simulink model "W01_Base_Map_cs"  (R2019a)
settings: Solver=FixedStepDiscrete  StartTime=0.0  StopTime=40  FixedStep=1/20  RelTol=1e-3
PreLoadFcn:
  | mbxruntime.callbacks.PreLoadFcn(bdroot);
  | check_NUTS_defined
  | model_closed = 0;
  | assignin('base',['model_closed_' bdroot],false);
PostLoadFcn:
  | mbxruntime.callbacks.PostLoadFcn(bdroot);
InitFcn:
  | mbxruntime.callbacks.InitFcn(bdroot);
StartFcn:
  | mbxruntime.callbacks.StartFcn(bdroot);
StopFcn:
  | mbxruntime.callbacks.StopFcn(bdroot);;
  | 
model workspace: external: MAT-File .\W01_Base_Map_cs_hws.mat (data not in the file)
undefined symbols (not defined in the file or in its folder): DiscIntNeverNeededParam, InitImageOutputDir, mbxruntime, tabledata, W01_Base_Map_cs_328ec7e3a8cd5b54, W01_Base_Map_cs_423c72fa17799c7f, W01_Base_Map_cs_514c2dea2cdbe680, W01_Base_Map_cs_51d6e6e467bedba1, W01_Base_Map_cs_563ebd29d1fd6c09, W01_Base_Map_cs_57ea59d0358dab77, W01_Base_Map_cs_669d1acb174df2b9, W01_Base_Map_cs_774a522413284ef7, W01_Base_Map_cs_9538d35a279fbe4e, W01_Base_Map_cs_9f504bb84aebc2fd, W01_Base_Map_cs_a242ed7539861165, W01_Base_Map_cs_ae41b72d7e14f81d, W01_Base_Map_cs_Audi_A8_Sedan_1_Path_pathUniqueID, W01_Base_Map_cs_b5931a786e299506, W01_Base_Map_cs_b7f45a070fa6e639, W01_Base_Map_cs_c02beb48492dde12, W01_Base_Map_cs_c75b75e9f6b035bf, W01_Base_Map_cs_cf83ac8e8b053cbf, W01_Base_Map_cs_Child_RegularAni_1_Path_pathUniqueID, W01_Base_Map_cs_Child_RegularAni_2_Path_pathUniqueID, W01_Base_Map_cs_Citroen_C3_Hatchback_1_Path_pathUniqueID, W01_Base_Map_cs_d4423fcf1c0d6fc4, W01_Base_Map_cs_df133aa86d9852fe, W01_Base_Map_cs_Female_RegularAni_1_Path_pathUniqueID, W01_Base_Map_cs_Male_RegularAni_1_Path_pathUniqueID, W01_Base_Map_cs_Male_RegularAni_2_Path_pathUniqueID
libraries: simulink_extras x41, adeye_lib x15, simulink x10, dspindex x6, PreScanSimulinkLibrary x4, sharedtransform x3, robotcorelib x1, PreScanUsefulBlocks x1
(part 10 of 11)

== system W01_Base_Map_cs/TrafficLightRoadSideNL_6/Orange_Mux ==
  MSCD [Cd] : Inport
  Position (xyz) [m] : Inport  Port=2
  Orientation (RPY) [deg] : Inport  Port=3
  Color [-] : Inport  Port=4
  TextureResourceID [-] : Inport  Port=5
  Bus Creator : BusCreator  Inputs='Intensity','Position','Orientation','Color','TextureResourceID'  OutDataTypeStr=Bus: PRESCAN_VISULIGHTACTUATOR_DATA  NonVirtualBus=on
  Bus Creator1 : BusCreator  Inputs=3  OutDataTypeStr=Bus: PRESCAN_RGB_DATA  NonVirtualBus=on
  Bus Creator2 : BusCreator  Inputs=3  OutDataTypeStr=Bus: PRESCAN_RPY_DATA  NonVirtualBus=on
  Bus Creator3 : BusCreator  Inputs=3  OutDataTypeStr=Bus: PRESCAN_XYZ_DATA  NonVirtualBus=on
  Data Type Conversion : DataTypeConversion  OutDataTypeStr=int32  RndMeth=Nearest
  Degrees to Radians : simulink_extras/Transformations/Degrees to Radians
  Demux : Demux  Outputs=3
  Demux1 : Demux  Outputs=3
  Demux2 : Demux  Outputs=3
  Lights : Outport
  wires:
  TextureResourceID [-]/1 -> Data Type Conversion/1  "TextureResourceID"
  MSCD [Cd]/1 -> Bus Creator/1  "Intensity"
  Bus Creator/1 -> Lights/1
  Demux/1 -> Bus Creator1/1  "R"
  Demux/2 -> Bus Creator1/2  "G"
  Demux/3 -> Bus Creator1/3  "B"
  Color [-]/1 -> Demux/1  "Color"
  Bus Creator1/1 -> Bus Creator/4  "Color"
  Demux1/1 -> Bus Creator2/1  "Roll"
  Demux1/2 -> Bus Creator2/2  "Pitch"
  Demux1/3 -> Bus Creator2/3  "Yaw"
  Orientation (RPY) [deg]/1 -> Degrees to Radians/1  "Orientation"
  Bus Creator2/1 -> Bus Creator/3  "Orientation"
  Demux2/1 -> Bus Creator3/1  "X"
  Demux2/2 -> Bus Creator3/2  "Y"
  Demux2/3 -> Bus Creator3/3  "Z"
  Position (xyz) [m]/1 -> Demux2/1  "Position"
  Bus Creator3/1 -> Bus Creator/2  "Position"
  Data Type Conversion/1 -> Bus Creator/5  "TextureResourceID"
  Degrees to Radians/1 -> Demux1/1

== system W01_Base_Map_cs/TrafficLightRoadSideNL_6/Red_Mux ==
  MSCD [Cd] : Inport
  Position (xyz) [m] : Inport  Port=2
  Orientation (RPY) [deg] : Inport  Port=3
  Color [-] : Inport  Port=4
  TextureResourceID [-] : Inport  Port=5
  Bus Creator : BusCreator  Inputs='Intensity','Position','Orientation','Color','TextureResourceID'  OutDataTypeStr=Bus: PRESCAN_VISULIGHTACTUATOR_DATA  NonVirtualBus=on
  Bus Creator1 : BusCreator  Inputs=3  OutDataTypeStr=Bus: PRESCAN_RGB_DATA  NonVirtualBus=on
  Bus Creator2 : BusCreator  Inputs=3  OutDataTypeStr=Bus: PRESCAN_RPY_DATA  NonVirtualBus=on
  Bus Creator3 : BusCreator  Inputs=3  OutDataTypeStr=Bus: PRESCAN_XYZ_DATA  NonVirtualBus=on
  Data Type Conversion : DataTypeConversion  OutDataTypeStr=int32  RndMeth=Nearest
  Degrees to Radians : simulink_extras/Transformations/Degrees to Radians
  Demux : Demux  Outputs=3
  Demux1 : Demux  Outputs=3
  Demux2 : Demux  Outputs=3
  Lights : Outport
  wires:
  TextureResourceID [-]/1 -> Data Type Conversion/1  "TextureResourceID"
  MSCD [Cd]/1 -> Bus Creator/1  "Intensity"
  Bus Creator/1 -> Lights/1
  Demux/1 -> Bus Creator1/1  "R"
  Demux/2 -> Bus Creator1/2  "G"
  Demux/3 -> Bus Creator1/3  "B"
  Color [-]/1 -> Demux/1  "Color"
  Bus Creator1/1 -> Bus Creator/4  "Color"
  Demux1/1 -> Bus Creator2/1  "Roll"
  Demux1/2 -> Bus Creator2/2  "Pitch"
  Demux1/3 -> Bus Creator2/3  "Yaw"
  Orientation (RPY) [deg]/1 -> Degrees to Radians/1  "Orientation"
  Bus Creator2/1 -> Bus Creator/3  "Orientation"
  Demux2/1 -> Bus Creator3/1  "X"
  Demux2/2 -> Bus Creator3/2  "Y"
  Demux2/3 -> Bus Creator3/3  "Z"
  Position (xyz) [m]/1 -> Demux2/1  "Position"
  Bus Creator3/1 -> Bus Creator/2  "Position"
  Data Type Conversion/1 -> Bus Creator/5  "TextureResourceID"
  Degrees to Radians/1 -> Demux1/1

== system W01_Base_Map_cs/TrafficLightRoadSideNL_7/Green_Mux ==
  MSCD [Cd] : Inport
  Position (xyz) [m] : Inport  Port=2
  Orientation (RPY) [deg] : Inport  Port=3
  Color [-] : Inport  Port=4
  TextureResourceID [-] : Inport  Port=5
  Bus Creator : BusCreator  Inputs='Intensity','Position','Orientation','Color','TextureResourceID'  OutDataTypeStr=Bus: PRESCAN_VISULIGHTACTUATOR_DATA  NonVirtualBus=on
  Bus Creator1 : BusCreator  Inputs=3  OutDataTypeStr=Bus: PRESCAN_RGB_DATA  NonVirtualBus=on
  Bus Creator2 : BusCreator  Inputs=3  OutDataTypeStr=Bus: PRESCAN_RPY_DATA  NonVirtualBus=on
  Bus Creator3 : BusCreator  Inputs=3  OutDataTypeStr=Bus: PRESCAN_XYZ_DATA  NonVirtualBus=on
  Data Type Conversion : DataTypeConversion  OutDataTypeStr=int32  RndMeth=Nearest
  Degrees to Radians : simulink_extras/Transformations/Degrees to Radians
  Demux : Demux  Outputs=3
  Demux1 : Demux  Outputs=3
  Demux2 : Demux  Outputs=3
  Lights : Outport
  wires:
  TextureResourceID [-]/1 -> Data Type Conversion/1  "TextureResourceID"
  MSCD [Cd]/1 -> Bus Creator/1  "Intensity"
  Bus Creator/1 -> Lights/1
  Demux/1 -> Bus Creator1/1  "R"
  Demux/2 -> Bus Creator1/2  "G"
  Demux/3 -> Bus Creator1/3  "B"
  Color [-]/1 -> Demux/1  "Color"
  Bus Creator1/1 -> Bus Creator/4  "Color"
  Demux1/1 -> Bus Creator2/1  "Roll"
  Demux1/2 -> Bus Creator2/2  "Pitch"
  Demux1/3 -> Bus Creator2/3  "Yaw"
  Orientation (RPY) [deg]/1 -> Degrees to Radians/1  "Orientation"
  Bus Creator2/1 -> Bus Creator/3  "Orientation"
  Demux2/1 -> Bus Creator3/1  "X"
  Demux2/2 -> Bus Creator3/2  "Y"
  Demux2/3 -> Bus Creator3/3  "Z"
  Position (xyz) [m]/1 -> Demux2/1  "Position"
  Bus Creator3/1 -> Bus Creator/2  "Position"
  Data Type Conversion/1 -> Bus Creator/5  "TextureResourceID"
  Degrees to Radians/1 -> Demux1/1

== system W01_Base_Map_cs/TrafficLightRoadSideNL_7/Orange_Mux ==
  MSCD [Cd] : Inport
  Position (xyz) [m] : Inport  Port=2
  Orientation (RPY) [deg] : Inport  Port=3
  Color [-] : Inport  Port=4
  TextureResourceID [-] : Inport  Port=5
  Bus Creator : BusCreator  Inputs='Intensity','Position','Orientation','Color','TextureResourceID'  OutDataTypeStr=Bus: PRESCAN_VISULIGHTACTUATOR_DATA  NonVirtualBus=on
  Bus Creator1 : BusCreator  Inputs=3  OutDataTypeStr=Bus: PRESCAN_RGB_DATA  NonVirtualBus=on
  Bus Creator2 : BusCreator  Inputs=3  OutDataTypeStr=Bus: PRESCAN_RPY_DATA  NonVirtualBus=on
  Bus Creator3 : BusCreator  Inputs=3  OutDataTypeStr=Bus: PRESCAN_XYZ_DATA  NonVirtualBus=on
  Data Type Conversion : DataTypeConversion  OutDataTypeStr=int32  RndMeth=Nearest
  Degrees to Radians : simulink_extras/Transformations/Degrees to Radians
  Demux : Demux  Outputs=3
  Demux1 : Demux  Outputs=3
  Demux2 : Demux  Outputs=3
  Lights : Outport
  wires:
  TextureResourceID [-]/1 -> Data Type Conversion/1  "TextureResourceID"
  MSCD [Cd]/1 -> Bus Creator/1  "Intensity"
  Bus Creator/1 -> Lights/1
  Demux/1 -> Bus Creator1/1  "R"
  Demux/2 -> Bus Creator1/2  "G"
  Demux/3 -> Bus Creator1/3  "B"
  Color [-]/1 -> Demux/1  "Color"
  Bus Creator1/1 -> Bus Creator/4  "Color"
  Demux1/1 -> Bus Creator2/1  "Roll"
  Demux1/2 -> Bus Creator2/2  "Pitch"
  Demux1/3 -> Bus Creator2/3  "Yaw"
  Orientation (RPY) [deg]/1 -> Degrees to Radians/1  "Orientation"
  Bus Creator2/1 -> Bus Creator/3  "Orientation"
  Demux2/1 -> Bus Creator3/1  "X"
  Demux2/2 -> Bus Creator3/2  "Y"
  Demux2/3 -> Bus Creator3/3  "Z"
  Position (xyz) [m]/1 -> Demux2/1  "Position"
  Bus Creator3/1 -> Bus Creator/2  "Position"
  Data Type Conversion/1 -> Bus Creator/5  "TextureResourceID"
  Degrees to Radians/1 -> Demux1/1

== system W01_Base_Map_cs/TrafficLightRoadSideNL_7/Red_Mux ==
  MSCD [Cd] : Inport
  Position (xyz) [m] : Inport  Port=2
  Orientation (RPY) [deg] : Inport  Port=3
  Color [-] : Inport  Port=4
  TextureResourceID [-] : Inport  Port=5
  Bus Creator : BusCreator  Inputs='Intensity','Position','Orientation','Color','TextureResourceID'  OutDataTypeStr=Bus: PRESCAN_VISULIGHTACTUATOR_DATA  NonVirtualBus=on
  Bus Creator1 : BusCreator  Inputs=3  OutDataTypeStr=Bus: PRESCAN_RGB_DATA  NonVirtualBus=on
  Bus Creator2 : BusCreator  Inputs=3  OutDataTypeStr=Bus: PRESCAN_RPY_DATA  NonVirtualBus=on
  Bus Creator3 : BusCreator  Inputs=3  OutDataTypeStr=Bus: PRESCAN_XYZ_DATA  NonVirtualBus=on
  Data Type Conversion : DataTypeConversion  OutDataTypeStr=int32  RndMeth=Nearest
  Degrees to Radians : simulink_extras/Transformations/Degrees to Radians
  Demux : Demux  Outputs=3
  Demux1 : Demux  Outputs=3
  Demux2 : Demux  Outputs=3
  Lights : Outport
  wires:
  TextureResourceID [-]/1 -> Data Type Conversion/1  "TextureResourceID"
  MSCD [Cd]/1 -> Bus Creator/1  "Intensity"
  Bus Creator/1 -> Lights/1
  Demux/1 -> Bus Creator1/1  "R"
  Demux/2 -> Bus Creator1/2  "G"
  Demux/3 -> Bus Creator1/3  "B"
  Color [-]/1 -> Demux/1  "Color"
  Bus Creator1/1 -> Bus Creator/4  "Color"
  Demux1/1 -> Bus Creator2/1  "Roll"
  Demux1/2 -> Bus Creator2/2  "Pitch"
  Demux1/3 -> Bus Creator2/3  "Yaw"
  Orientation (RPY) [deg]/1 -> Degrees to Radians/1  "Orientation"
  Bus Creator2/1 -> Bus Creator/3  "Orientation"
  Demux2/1 -> Bus Creator3/1  "X"
  Demux2/2 -> Bus Creator3/2  "Y"
  Demux2/3 -> Bus Creator3/3  "Z"
  Position (xyz) [m]/1 -> Demux2/1  "Position"
  Bus Creator3/1 -> Bus Creator/2  "Position"
  Data Type Conversion/1 -> Bus Creator/5  "TextureResourceID"
  Degrees to Radians/1 -> Demux1/1

== system W01_Base_Map_cs/TrafficLightRoadSideNL_8/Green_Mux ==
  MSCD [Cd] : Inport
  Position (xyz) [m] : Inport  Port=2
  Orientation (RPY) [deg] : Inport  Port=3
  Color [-] : Inport  Port=4
  TextureResourceID [-] : Inport  Port=5
  Bus Creator : BusCreator  Inputs='Intensity','Position','Orientation','Color','TextureResourceID'  OutDataTypeStr=Bus: PRESCAN_VISULIGHTACTUATOR_DATA  NonVirtualBus=on
  Bus Creator1 : BusCreator  Inputs=3  OutDataTypeStr=Bus: PRESCAN_RGB_DATA  NonVirtualBus=on
  Bus Creator2 : BusCreator  Inputs=3  OutDataTypeStr=Bus: PRESCAN_RPY_DATA  NonVirtualBus=on
  Bus Creator3 : BusCreator  Inputs=3  OutDataTypeStr=Bus: PRESCAN_XYZ_DATA  NonVirtualBus=on
  Data Type Conversion : DataTypeConversion  OutDataTypeStr=int32  RndMeth=Nearest
  Degrees to Radians : simulink_extras/Transformations/Degrees to Radians
  Demux : Demux  Outputs=3
  Demux1 : Demux  Outputs=3
  Demux2 : Demux  Outputs=3
  Lights : Outport
  wires:
  TextureResourceID [-]/1 -> Data Type Conversion/1  "TextureResourceID"
  MSCD [Cd]/1 -> Bus Creator/1  "Intensity"
  Bus Creator/1 -> Lights/1
  Demux/1 -> Bus Creator1/1  "R"
  Demux/2 -> Bus Creator1/2  "G"
  Demux/3 -> Bus Creator1/3  "B"
  Color [-]/1 -> Demux/1  "Color"
  Bus Creator1/1 -> Bus Creator/4  "Color"
  Demux1/1 -> Bus Creator2/1  "Roll"
  Demux1/2 -> Bus Creator2/2  "Pitch"
  Demux1/3 -> Bus Creator2/3  "Yaw"
  Orientation (RPY) [deg]/1 -> Degrees to Radians/1  "Orientation"
  Bus Creator2/1 -> Bus Creator/3  "Orientation"
  Demux2/1 -> Bus Creator3/1  "X"
  Demux2/2 -> Bus Creator3/2  "Y"
  Demux2/3 -> Bus Creator3/3  "Z"
  Position (xyz) [m]/1 -> Demux2/1  "Position"
  Bus Creator3/1 -> Bus Creator/2  "Position"
  Data Type Conversion/1 -> Bus Creator/5  "TextureResourceID"
  Degrees to Radians/1 -> Demux1/1

== system W01_Base_Map_cs/TrafficLightRoadSideNL_8/Orange_Mux ==
  MSCD [Cd] : Inport
  Position (xyz) [m] : Inport  Port=2
  Orientation (RPY) [deg] : Inport  Port=3
  Color [-] : Inport  Port=4
  TextureResourceID [-] : Inport  Port=5
  Bus Creator : BusCreator  Inputs='Intensity','Position','Orientation','Color','TextureResourceID'  OutDataTypeStr=Bus: PRESCAN_VISULIGHTACTUATOR_DATA  NonVirtualBus=on
  Bus Creator1 : BusCreator  Inputs=3  OutDataTypeStr=Bus: PRESCAN_RGB_DATA  NonVirtualBus=on
  Bus Creator2 : BusCreator  Inputs=3  OutDataTypeStr=Bus: PRESCAN_RPY_DATA  NonVirtualBus=on
  Bus Creator3 : BusCreator  Inputs=3  OutDataTypeStr=Bus: PRESCAN_XYZ_DATA  NonVirtualBus=on
  Data Type Conversion : DataTypeConversion  OutDataTypeStr=int32  RndMeth=Nearest
  Degrees to Radians : simulink_extras/Transformations/Degrees to Radians
  Demux : Demux  Outputs=3
  Demux1 : Demux  Outputs=3
  Demux2 : Demux  Outputs=3
  Lights : Outport
  wires:
  TextureResourceID [-]/1 -> Data Type Conversion/1  "TextureResourceID"
  MSCD [Cd]/1 -> Bus Creator/1  "Intensity"
  Bus Creator/1 -> Lights/1
  Demux/1 -> Bus Creator1/1  "R"
  Demux/2 -> Bus Creator1/2  "G"
  Demux/3 -> Bus Creator1/3  "B"
  Color [-]/1 -> Demux/1  "Color"
  Bus Creator1/1 -> Bus Creator/4  "Color"
  Demux1/1 -> Bus Creator2/1  "Roll"
  Demux1/2 -> Bus Creator2/2  "Pitch"
  Demux1/3 -> Bus Creator2/3  "Yaw"
  Orientation (RPY) [deg]/1 -> Degrees to Radians/1  "Orientation"
  Bus Creator2/1 -> Bus Creator/3  "Orientation"
  Demux2/1 -> Bus Creator3/1  "X"
  Demux2/2 -> Bus Creator3/2  "Y"
  Demux2/3 -> Bus Creator3/3  "Z"
  Position (xyz) [m]/1 -> Demux2/1  "Position"
  Bus Creator3/1 -> Bus Creator/2  "Position"
  Data Type Conversion/1 -> Bus Creator/5  "TextureResourceID"
  Degrees to Radians/1 -> Demux1/1

== system W01_Base_Map_cs/TrafficLightRoadSideNL_8/Red_Mux ==
  MSCD [Cd] : Inport
  Position (xyz) [m] : Inport  Port=2
  Orientation (RPY) [deg] : Inport  Port=3
  Color [-] : Inport  Port=4
  TextureResourceID [-] : Inport  Port=5
  Bus Creator : BusCreator  Inputs='Intensity','Position','Orientation','Color','TextureResourceID'  OutDataTypeStr=Bus: PRESCAN_VISULIGHTACTUATOR_DATA  NonVirtualBus=on
  Bus Creator1 : BusCreator  Inputs=3  OutDataTypeStr=Bus: PRESCAN_RGB_DATA  NonVirtualBus=on
  Bus Creator2 : BusCreator  Inputs=3  OutDataTypeStr=Bus: PRESCAN_RPY_DATA  NonVirtualBus=on
  Bus Creator3 : BusCreator  Inputs=3  OutDataTypeStr=Bus: PRESCAN_XYZ_DATA  NonVirtualBus=on
  Data Type Conversion : DataTypeConversion  OutDataTypeStr=int32  RndMeth=Nearest
  Degrees to Radians : simulink_extras/Transformations/Degrees to Radians
  Demux : Demux  Outputs=3
  Demux1 : Demux  Outputs=3
  Demux2 : Demux  Outputs=3
  Lights : Outport
  wires:
  TextureResourceID [-]/1 -> Data Type Conversion/1  "TextureResourceID"
  MSCD [Cd]/1 -> Bus Creator/1  "Intensity"
  Bus Creator/1 -> Lights/1
  Demux/1 -> Bus Creator1/1  "R"
  Demux/2 -> Bus Creator1/2  "G"
  Demux/3 -> Bus Creator1/3  "B"
  Color [-]/1 -> Demux/1  "Color"
  Bus Creator1/1 -> Bus Creator/4  "Color"
  Demux1/1 -> Bus Creator2/1  "Roll"
  Demux1/2 -> Bus Creator2/2  "Pitch"
  Demux1/3 -> Bus Creator2/3  "Yaw"
  Orientation (RPY) [deg]/1 -> Degrees to Radians/1  "Orientation"
  Bus Creator2/1 -> Bus Creator/3  "Orientation"
  Demux2/1 -> Bus Creator3/1  "X"
  Demux2/2 -> Bus Creator3/2  "Y"
  Demux2/3 -> Bus Creator3/3  "Z"
  Position (xyz) [m]/1 -> Demux2/1  "Position"
  Bus Creator3/1 -> Bus Creator/2  "Position"
  Data Type Conversion/1 -> Bus Creator/5  "TextureResourceID"
  Degrees to Radians/1 -> Demux1/1

== system W01_Base_Map_cs/pose_otheCar/PoseArray Publisher ==
  seq : Inport
  frameId : Inport  Port=2
  frameId_length : Inport  Port=3
  poses : Inport  Port=4
  poses_length : Inport  Port=5
  seq1 : Inport  Port=6
  frameId1 : Inport  Port=7
  frameId_length1 : Inport  Port=8
  poses1 : Inport  Port=9
  poses_length1 : Inport  Port=10
  seq2 : Inport  Port=11
  frameId2 : Inport  Port=12
  frameId_length2 : Inport  Port=13
  poses2 : Inport  Port=14
  poses_length2 : Inport  Port=15
  Demux : Demux  Outputs=7
  Demux1 : Demux  Outputs=7
  Demux2 : Demux  Outputs=7
  S-Function Builder : S-Function  InitFcn=try, set_param(gcb,'FunctionName','PoseArray3_publisher'), end  FunctionName=PoseArray3_publisher  Parameters=int8(topic),int8(message_type),port,timeout  SFunctionModules=PoseArray3_publisher_wrapper rosbridge_functions  SFunctionDeploymentMode=off  EnableBusSupport=off  mask(S-Function Builder){}
      mask help: Simulink:masks:SFunctionBuilder_MD
      mask init:
      | val = [[.9  0.75 0.75 1 1 .9 .9 1]',[1 1 0.75 0.75 .9 .9 1 .9]'];try , sys = get_param(gcb,'SfunBuilderFcnName');if isempty(sys), sys = get_param(gcb,'FunctionName'); end,catch, sys = get_param(gcb,'FunctionName'); end
      settings: CopyFcn=set_param(gcbh,'LinkStatus','none')  PreSaveFcn=try, set_param(gcb,'FunctionName','PoseArray3_publisher'), end  OpenFcn=sfunctionwizard(gcbh)
      mask Display: plot(val(:,1),val(:,2)),disp(sys), port_label('input',1,'seq'), port_label('input',2,'frameId'), port_label('input',3,'frameId_length'), port_label('input',4,'positionX'), port_label('input',5,'positionY'), port_label('input',6,'positionZ'), port_label('input',7,'orientationW'), port_label('input',8,'orientationX'), port_label('input',9,'orientationY'), port_label('input',10,'orientationZ'), port_label('input',11,'poses_length'), port_label('input',12,'seq1'), port_label('input',13,'frameId1'), port_label('input',14,'frameId_length1'), port_label('input',15,'positionX1'), port_label('input',16,'positionY1'), port_label('input',17,'positionZ1'), port_label('input',18,'orientationW1'), port_label('input',19,'orientationX1'), port_label('input',20,'orientationY1'), port_label('input',21,'orientationZ1'), port_label('input',22,'poses_length1'), port_label('input',23,'seq2'), port_label('input',24,'frameId2'), port_label('input',25,'frameId_length2'), port_label('input',26,'positionX2'), port_label('input',27,'positionY2'), port_label('input',28,'positionZ2'), port_label('input',29,'orientationW2'), port_label('input',30,'orientationX2'), port_label('input',31,'orientationY2'), port_label('input',32,'orientationZ2'), port_label('input',33,'poses_length2')
  wires:
  seq/1 -> S-Function Builder/1
  Demux/1 -> S-Function Builder/4
  Demux/2 -> S-Function Builder/5
  Demux/3 -> S-Function Builder/6
  Demux/4 -> S-Function Builder/7
  Demux/5 -> S-Function Builder/8
  Demux/6 -> S-Function Builder/9
  Demux/7 -> S-Function Builder/10
  frameId_length/1 -> S-Function Builder/3
  frameId/1 -> S-Function Builder/2
  poses/1 -> Demux/1
  poses_length/1 -> S-Function Builder/11
  frameId1/1 -> S-Function Builder/13
  frameId_length1/1 -> S-Function Builder/14
  seq1/1 -> S-Function Builder/12
  Demux1/6 -> S-Function Builder/20
  Demux1/2 -> S-Function Builder/16
  Demux1/7 -> S-Function Builder/21
  Demux1/5 -> S-Function Builder/19
  Demux1/3 -> S-Function Builder/17
  Demux1/4 -> S-Function Builder/18
  Demux1/1 -> S-Function Builder/15
  poses1/1 -> Demux1/1
  poses_length1/1 -> S-Function Builder/22
  seq2/1 -> S-Function Builder/23
  frameId2/1 -> S-Function Builder/24
  frameId_length2/1 -> S-Function Builder/25
  Demux2/6 -> S-Function Builder/31
  Demux2/4 -> S-Function Builder/29
  Demux2/3 -> S-Function Builder/28
  Demux2/2 -> S-Function Builder/27
  Demux2/7 -> S-Function Builder/32
  poses2/1 -> Demux2/1
  Demux2/1 -> S-Function Builder/26
  Demux2/5 -> S-Function Builder/30
  poses_length2/1 -> S-Function Builder/33

== system W01_Base_Map_cs/Audi_A8_Sedan_1/SELF_Demux/compas converter ==
  rotz [rad] : Inport
  cart2compas : Subsystem
  rad2deg : Gain  Gain=180/pi
  heading [deg] : Outport
  wires:
  rad2deg/1 -> cart2compas/1(Angle [deg])
  rotz [rad]/1 -> rad2deg/1
  cart2compas/1(heading [deg]) -> heading [deg]/1

== system W01_Base_Map_cs/BMW_X5_SUV_1/Dynamics_Empty/MuxState ==
  note: mode: Dynamics
  note: mode: Positioning
  note: mode: Dynamics
      | VelVEHICLE
      | wrt VEH
  note: AnglesVEHICLE
      | wrtGLOB
  note: For state mode 'Dynamic' positions
      | are not taken into account, as they
      | are computed by integrating velocity.
      | Click annotation for Help.
  x [m] : Inport  SampleTime=TimeStep
  y [m] : Inport  Port=2  SampleTime=TimeStep
  z [m] : Inport  Port=3  SampleTime=TimeStep
  dx [m/s] : Inport  Port=4  SampleTime=TimeStep
  dy [m/s] : Inport  Port=5  SampleTime=TimeStep
  dz [m/s] : Inport  Port=6  SampleTime=TimeStep
  R [rad] : Inport  Port=7  SampleTime=TimeStep
  P [rad] : Inport  Port=8  SampleTime=TimeStep
  Y [rad] : Inport  Port=9  SampleTime=TimeStep
  Constant : Constant  DisableCoverage=on  Value=positioningmode
  Discrete-Time Integrator : DiscreteIntegrator  SampleTime=TimeStep  ICPrevOutput=DiscIntNeverNeededParam  ICPrevScaledInput=DiscIntNeverNeededParam
  Ground : Ground
  Ground1 : Ground
  Mux1 : Mux  Inputs=[3 3]
  Mux2 : Mux  Inputs=3
  Mux3 : Mux  Inputs=3
  Mux4 : Mux  Inputs=3
  Mux5 : Mux  Inputs=[3 3]
  Mux6 : Mux  Inputs=[6 3]
  Switch : Switch  Threshold=0.5
  Transformation_BODY2GLOBAL : PreScanSimulinkLibrary/Simple_Vehicle_Dynamics/Chassis/MuxDynState/Transformation_BODY2GLOBAL  SystemSampleTime=-1
  mux3 : Mux  Inputs=3
  state : Outport
  wires:
  Constant/1 -> Switch/2
  Mux6/1 -> state/1
  Mux4/1 -> Mux1/1
  Mux5/1 -> Switch/3
  Mux1/1 -> Switch/1
  Switch/1 -> Mux6/1  "PosVeh wrt  GLOB"
  P [rad]/1 -> Mux3/2
  R [rad]/1 -> Mux3/1
  dz [m/s]/1 -> Mux2/3
  dy [m/s]/1 -> Mux2/2
  dx [m/s]/1 -> Mux2/1
  z [m]/1 -> Mux4/3
  y [m]/1 -> Mux4/2
  x [m]/1 -> Mux4/1
  Ground1/1 -> mux3/2  "pitch"
  Y [rad]/1 -> mux3/3, Mux3/3  "yaw"
  Mux3/1 -> Mux6/2
  Transformation_BODY2GLOBAL/1 -> Discrete-Time Integrator/1, Mux5/2  "VelVEH wrt  GLOB"
  mux3/1 -> Transformation_BODY2GLOBAL/2
  Ground/1 -> mux3/1  "roll"
  Mux2/1 -> Mux1/2, Transformation_BODY2GLOBAL/1
  Discrete-Time Integrator/1 -> Mux5/1  "PosVEH wrt  GLOB"

== system W01_Base_Map_cs/BMW_X5_SUV_1/Dynamics_Empty/STATE_BMW_X5_SUV_1 ==
  State : Inport  SampleTime=TimeStep
  Bus Creator : BusCreator  Inputs=15  OutDataTypeStr=Bus: PRESCAN_STATEACTUATORDATA  NonVirtualBus=on
  Constant : Constant  Value=0
  Demux : Demux  Outputs=15
  Mux : Mux  Inputs=3
  Mux1 : Mux  Inputs=3
  Mux2 : Mux  Inputs=3
  iniBODYAngles wrtVEH [rad] : Constant  Value=Roll0  SampleTime=TimeStep
  iniBODYAngles wrtVEH [rad]1 : Constant  Value=Pitch0  SampleTime=TimeStep
  iniVEHAngles wrtGLOB [rad] : Constant  Value=Yaw0  SampleTime=TimeStep
  iniVEHposition wrtGLOB [m] : Constant  Value=x0  SampleTime=TimeStep
  iniVEHposition wrtGLOB [m]1 : Constant  Value=y0  SampleTime=TimeStep
  iniVEHposition wrtGLOB [m]2 : Constant  Value=z0  SampleTime=TimeStep
  state2FullState : PreScanSimulinkLibrary/state2FullState  SystemSampleTime=-1
  StateBus : Outport  OutDataTypeStr=Bus: PRESCAN_STATEACTUATORDATA
  wires:
  Mux2/1 -> state2FullState/4
  iniVEHAngles wrtGLOB [rad]/1 -> Mux2/3
  Mux1/1 -> state2FullState/3
  Constant/1 -> Mux2/1, Mux2/2, Mux1/3
  iniBODYAngles wrtVEH [rad]1/1 -> Mux1/2
  iniBODYAngles wrtVEH [rad]/1 -> Mux1/1
  Mux/1 -> state2FullState/2
  iniVEHposition wrtGLOB [m]2/1 -> Mux/3
  iniVEHposition wrtGLOB [m]/1 -> Mux/1
  iniVEHposition wrtGLOB [m]1/1 -> Mux/2
  Demux/15 -> Bus Creator/15  "AngularVelocityYaw"
  Demux/14 -> Bus Creator/14  "AngularVelocityPitch"
  Demux/13 -> Bus Creator/13  "AngularVelocityRoll"
  Demux/12 -> Bus Creator/12  "OrientationYaw"
  Demux/11 -> Bus Creator/11  "OrientationPitch"
  Demux/10 -> Bus Creator/10  "OrientationRoll"
  Demux/9 -> Bus Creator/9  "AccelerationZ"
  Demux/8 -> Bus Creator/8  "AccelerationY"
  Demux/7 -> Bus Creator/7  "AccelerationX"
  Demux/6 -> Bus Creator/6  "VelocityZ"
  Demux/5 -> Bus Creator/5  "VelocityY"
  Demux/4 -> Bus Creator/4  "VelocityX"
  Demux/3 -> Bus Creator/3  "PositionZ"
  Demux/2 -> Bus Creator/2  "PositionY"
  Demux/1 -> Bus Creator/1  "PositionX"
  state2FullState/1 -> Demux/1
  State/1 -> state2FullState/1
  Bus Creator/1 -> StateBus/1

== system W01_Base_Map_cs/BMW_X5_SUV_1/Dynamics_Empty/Subsystem1 ==
  note: For state mode 'Dynamic' positions
      | are not taken into account, as they
      | are computed by integrating velocity.
      | Click annotation for Help.
  In1 : Inport
  Data Type Conversion{6..11} (6 alike) : DataTypeConversion
  Discrete-Time Integrator4 : DiscreteIntegrator  SampleTime=-1  ICPrevOutput=DiscIntNeverNeededParam  ICPrevScaledInput=DiscIntNeverNeededParam
  Discrete-Time Integrator5 : DiscreteIntegrator  SampleTime=-1  ICPrevOutput=DiscIntNeverNeededParam  ICPrevScaledInput=DiscIntNeverNeededParam
  Discrete-Time Integrator6 : DiscreteIntegrator  SampleTime=-1  ICPrevOutput=DiscIntNeverNeededParam  ICPrevScaledInput=DiscIntNeverNeededParam
  Subsystem : Subsystem
  TwistStamped Subscriber : Subsystem  mask{topic='/TwistS', message_type='geometry_msgs/TwistStamped', port=9090, timeout=2}
      mask prompts: topic "Topic name"; message_type "Message type"; timeout "Timeout (s)"
  Out1 : Outport
  Out2 : Outport  Port=2
  Out3 : Outport  Port=3
  Out4 : Outport  Port=4
  Out5 : Outport  Port=5
  Out6 : Outport  Port=6
  wires:
  Discrete-Time Integrator6/1 -> Out4/1
  In1/1 -> Subsystem/1(In1)
  Subsystem/1(Out1) -> Out1/1
  Data Type Conversion8/1 -> Out3/1
  Discrete-Time Integrator4/1 -> Out6/1
  Data Type Conversion7/1 -> Out2/1
  Discrete-Time Integrator5/1 -> Out5/1
  Data Type Conversion9/1 -> Discrete-Time Integrator6/1
  Data Type Conversion10/1 -> Discrete-Time Integrator5/1
  Data Type Conversion11/1 -> Discrete-Time Integrator4/1
  Data Type Conversion6/1 -> Subsystem/2(In2)
  TwistStamped Subscriber/1(linear_x) -> Data Type Conversion6/1
  TwistStamped Subscriber/2(linear_y) -> Data Type Conversion7/1
  TwistStamped Subscriber/3(linear_z) -> Data Type Conversion8/1
  TwistStamped Subscriber/4(angular_x) -> Data Type Conversion9/1
  TwistStamped Subscriber/5(angular_y) -> Data Type Conversion10/1
  TwistStamped Subscriber/6(angular_z) -> Data Type Conversion11/1

== system W01_Base_Map_cs/BMW_X5_SUV_1/Fault Injection Camera1/If Action Subsystem ==
  In1 : Inport
  In2 : Inport  Port=2
  In3 : Inport  Port=3
  Action Port : ActionPort
  Out1 : Outport
  Out2 : Outport  Port=2
  Out3 : Outport  Port=3
  wires:
  In1/1 -> Out1/1
  In2/1 -> Out2/1
  In3/1 -> Out3/1

== system W01_Base_Map_cs/BMW_X5_SUV_1/Fault Injection Camera1/If Action Subsystem1 ==
  In2 : Inport
  In3 : Inport  Port=2
  In4 : Inport  Port=3
  In5 : Inport  Port=4
  In6 : Inport  Port=5
  In7 : Inport  Port=6
  Action Port : ActionPort
  Assignment1 : Assignment  NumberOfDimensions=2  DiagnosticForDimensions=Warning  IndexOptions=Starting index (port),Starting index (port)  Indices=1,1  OutputSizes=1000,1
  Assignment2 : Assignment  NumberOfDimensions=2  DiagnosticForDimensions=Warning  IndexOptions=Starting index (port),Starting index (port)  Indices=1,1  OutputSizes=1000,1
  Assignment3 : Assignment  NumberOfDimensions=2  DiagnosticForDimensions=Warning  IndexOptions=Starting index (port),Starting index (port)  Indices=1,1  OutputSizes=1000,1
  Out2 : Outport
  Out3 : Outport  Port=2
  Out4 : Outport  Port=3
  wires:
  In2/1 -> Assignment3/3, Assignment1/3, Assignment2/3
  In6/1 -> Assignment1/1
  Assignment1/1 -> Out3/1
  In4/1 -> Assignment3/2, Assignment1/2, Assignment2/2
  Assignment2/1 -> Out2/1
  Assignment3/1 -> Out4/1
  In7/1 -> Assignment3/1
  In5/1 -> Assignment2/1
  In3/1 -> Assignment2/4, Assignment1/4, Assignment3/4

== system W01_Base_Map_cs/BMW_X5_SUV_1/Fault Injection Listener Camera 1/Int16 Subscriber ==
  S-Function Builder : S-Function  InitFcn=try, set_param(gcb,'FunctionName','int16_subscriber'), end  FunctionName=int16_subscriber  Parameters=int8(topic),int8(message_type),port,timeout  SFunctionModules=int16_subscriber_wrapper rosbridge_functions  SFunctionDeploymentMode=off  EnableBusSupport=off  mask(S-Function Builder){}
      mask help: Simulink:masks:SFunctionBuilder_MD
      mask init: same as W01_Base_Map_cs/pose_otheCar/PoseArray Publisher/S-Function Builder
      settings: CopyFcn=set_param(gcbh,'LinkStatus','none')  PreSaveFcn=try, set_param(gcb,'FunctionName','int16_subscriber'), end  OpenFcn=sfunctionwizard(gcbh)
      mask Display: plot(val(:,1),val(:,2)),disp(sys), port_label('output',1,'data')
  data : Outport
  wires:
  S-Function Builder/1 -> data/1

== system W01_Base_Map_cs/BMW_X5_SUV_1/Fault Injection Listener Camera 2/Int16 Subscriber ==
  S-Function Builder : S-Function  InitFcn=try, set_param(gcb,'FunctionName','int16_subscriber'), end  FunctionName=int16_subscriber  Parameters=int8(topic),int8(message_type),port,timeout  SFunctionModules=int16_subscriber_wrapper rosbridge_functions  SFunctionDeploymentMode=off  EnableBusSupport=off  mask(S-Function Builder){}
      mask help: Simulink:masks:SFunctionBuilder_MD
      mask init: same as W01_Base_Map_cs/pose_otheCar/PoseArray Publisher/S-Function Builder
      settings: CopyFcn=set_param(gcbh,'LinkStatus','none')  PreSaveFcn=try, set_param(gcb,'FunctionName','int16_subscriber'), end  OpenFcn=sfunctionwizard(gcbh)
      mask Display: plot(val(:,1),val(:,2)),disp(sys), port_label('output',1,'data')
  data : Outport
  wires:
  S-Function Builder/1 -> data/1

== system W01_Base_Map_cs/BMW_X5_SUV_1/Fault Injection Listener GNSS/Int16 Subscriber ==
  S-Function Builder : S-Function  InitFcn=try, set_param(gcb,'FunctionName','int16_subscriber'), end  FunctionName=int16_subscriber  Parameters=int8(topic),int8(message_type),port,timeout  SFunctionModules=int16_subscriber_wrapper rosbridge_functions  SFunctionDeploymentMode=off  EnableBusSupport=off  mask(S-Function Builder){}
      mask help: Simulink:masks:SFunctionBuilder_MD
      mask init: same as W01_Base_Map_cs/pose_otheCar/PoseArray Publisher/S-Function Builder
      settings: CopyFcn=set_param(gcbh,'LinkStatus','none')  PreSaveFcn=try, set_param(gcb,'FunctionName','int16_subscriber'), end  OpenFcn=sfunctionwizard(gcbh)
      mask Display: plot(val(:,1),val(:,2)),disp(sys), port_label('output',1,'data')
  data : Outport
  wires:
  S-Function Builder/1 -> data/1

== system W01_Base_Map_cs/BMW_X5_SUV_1/Fault Injection Listener Lidar 1/Int16 Subscriber ==
  S-Function Builder : S-Function  InitFcn=try, set_param(gcb,'FunctionName','int16_subscriber'), end  FunctionName=int16_subscriber  Parameters=int8(topic),int8(message_type),port,timeout  SFunctionModules=int16_subscriber_wrapper rosbridge_functions  SFunctionDeploymentMode=off  EnableBusSupport=off  mask(S-Function Builder){}
      mask help: Simulink:masks:SFunctionBuilder_MD
      mask init: same as W01_Base_Map_cs/pose_otheCar/PoseArray Publisher/S-Function Builder
      settings: CopyFcn=set_param(gcbh,'LinkStatus','none')  PreSaveFcn=try, set_param(gcb,'FunctionName','int16_subscriber'), end  OpenFcn=sfunctionwizard(gcbh)
      mask Display: plot(val(:,1),val(:,2)),disp(sys), port_label('output',1,'data')
  data : Outport
  wires:
  S-Function Builder/1 -> data/1

== system W01_Base_Map_cs/BMW_X5_SUV_1/Fault Injection Listener Lidar 2/Int16 Subscriber ==
  S-Function Builder : S-Function  InitFcn=try, set_param(gcb,'FunctionName','int16_subscriber'), end  FunctionName=int16_subscriber  Parameters=int8(topic),int8(message_type),port,timeout  SFunctionModules=int16_subscriber_wrapper rosbridge_functions  SFunctionDeploymentMode=off  EnableBusSupport=off  mask(S-Function Builder){}
      mask help: Simulink:masks:SFunctionBuilder_MD
      mask init: same as W01_Base_Map_cs/pose_otheCar/PoseArray Publisher/S-Function Builder
      settings: CopyFcn=set_param(gcbh,'LinkStatus','none')  PreSaveFcn=try, set_param(gcb,'FunctionName','int16_subscriber'), end  OpenFcn=sfunctionwizard(gcbh)
      mask Display: plot(val(:,1),val(:,2)),disp(sys), port_label('output',1,'data')
  data : Outport
  wires:
  S-Function Builder/1 -> data/1

== system W01_Base_Map_cs/BMW_X5_SUV_1/Fault Injection Listener Lidar 3/Int16 Subscriber ==
  S-Function Builder : S-Function  InitFcn=try, set_param(gcb,'FunctionName','int16_subscriber'), end  FunctionName=int16_subscriber  Parameters=int8(topic),int8(message_type),port,timeout  SFunctionModules=int16_subscriber_wrapper rosbridge_functions  SFunctionDeploymentMode=off  EnableBusSupport=off  mask(S-Function Builder){}
      mask help: Simulink:masks:SFunctionBuilder_MD
      mask init: same as W01_Base_Map_cs/pose_otheCar/PoseArray Publisher/S-Function Builder
      settings: CopyFcn=set_param(gcbh,'LinkStatus','none')  PreSaveFcn=try, set_param(gcb,'FunctionName','int16_subscriber'), end  OpenFcn=sfunctionwizard(gcbh)
      mask Display: plot(val(:,1),val(:,2)),disp(sys), port_label('output',1,'data')
  data : Outport
  wires:
  S-Function Builder/1 -> data/1

== system W01_Base_Map_cs/BMW_X5_SUV_1/Fault Injection Listener Lidar 4/Int16 Subscriber ==
  S-Function Builder : S-Function  InitFcn=try, set_param(gcb,'FunctionName','int16_subscriber'), end  FunctionName=int16_subscriber  Parameters=int8(topic),int8(message_type),port,timeout  SFunctionModules=int16_subscriber_wrapper rosbridge_functions  SFunctionDeploymentMode=off  EnableBusSupport=off  mask(S-Function Builder){}
      mask help: Simulink:masks:SFunctionBuilder_MD
      mask init: same as W01_Base_Map_cs/pose_otheCar/PoseArray Publisher/S-Function Builder
      settings: CopyFcn=set_param(gcbh,'LinkStatus','none')  PreSaveFcn=try, set_param(gcb,'FunctionName','int16_subscriber'), end  OpenFcn=sfunctionwizard(gcbh)
      mask Display: plot(val(:,1),val(:,2)),disp(sys), port_label('output',1,'data')
  data : Outport
  wires:
  S-Function Builder/1 -> data/1

== system W01_Base_Map_cs/BMW_X5_SUV_1/Fault Injection Listener Radar/Int16 Subscriber ==
  S-Function Builder : S-Function  InitFcn=try, set_param(gcb,'FunctionName','int16_subscriber'), end  FunctionName=int16_subscriber  Parameters=int8(topic),int8(message_type),port,timeout  SFunctionModules=int16_subscriber_wrapper rosbridge_functions  SFunctionDeploymentMode=off  EnableBusSupport=off  mask(S-Function Builder){}
      mask help: Simulink:masks:SFunctionBuilder_MD
      mask init: same as W01_Base_Map_cs/pose_otheCar/PoseArray Publisher/S-Function Builder
      settings: CopyFcn=set_param(gcbh,'LinkStatus','none')  PreSaveFcn=try, set_param(gcb,'FunctionName','int16_subscriber'), end  OpenFcn=sfunctionwizard(gcbh)
      mask Display: plot(val(:,1),val(:,2)),disp(sys), port_label('output',1,'data')
  data : Outport
  wires:
  S-Function Builder/1 -> data/1

== system W01_Base_Map_cs/BMW_X5_SUV_1/Fault Injection Listener TL Camera/Int16 Subscriber ==
  S-Function Builder : S-Function  InitFcn=try, set_param(gcb,'FunctionName','int16_subscriber'), end  FunctionName=int16_subscriber  Parameters=int8(topic),int8(message_type),port,timeout  SFunctionModules=int16_subscriber_wrapper rosbridge_functions  SFunctionDeploymentMode=off  EnableBusSupport=off  mask(S-Function Builder){}
      mask help: Simulink:masks:SFunctionBuilder_MD
      mask init: same as W01_Base_Map_cs/pose_otheCar/PoseArray Publisher/S-Function Builder
      settings: CopyFcn=set_param(gcbh,'LinkStatus','none')  PreSaveFcn=try, set_param(gcb,'FunctionName','int16_subscriber'), end  OpenFcn=sfunctionwizard(gcbh)
      mask Display: plot(val(:,1),val(:,2)),disp(sys), port_label('output',1,'data')
  data : Outport
  wires:
  S-Function Builder/1 -> data/1

== system W01_Base_Map_cs/BMW_X5_SUV_1/ROS Send Camera/Image Publisher1 ==
  height : Inport
  width : Inport  Port=2
  encoding_length : Inport  Port=3
  step : Inport  Port=4
  data : Inport  Port=5
  data_length : Inport  Port=6
  frameId_length : Inport  Port=7
  S-Function Builder : S-Function  InitFcn=try, set_param(gcb,'FunctionName','Image_publisher'), end  FunctionName=Image_publisher  Parameters=int8(topic),int8(message_type),int8(frame_id),port,timeout  SFunctionModules=Image_publisher_wrapper rosbridge_functions  SFunctionDeploymentMode=off  EnableBusSupport=off  mask(S-Function Builder){}
      mask help: Simulink:masks:SFunctionBuilder_MD
      mask init: same as W01_Base_Map_cs/pose_otheCar/PoseArray Publisher/S-Function Builder
      settings: CopyFcn=set_param(gcbh,'LinkStatus','none')  PreSaveFcn=try, set_param(gcb,'FunctionName','Image_publisher'), end  OpenFcn=sfunctionwizard(gcbh)
      mask Display: plot(val(:,1),val(:,2)),disp(sys), port_label('input',1,'height'), port_label('input',2,'width'), port_label('input',3,'encoding_length'), port_label('input',4,'step'), port_label('input',5,'data'), port_label('input',6,'data_length'), port_label('input',7,'frameId_length')
  wires:
  height/1 -> S-Function Builder/1
  width/1 -> S-Function Builder/2
  encoding_length/1 -> S-Function Builder/3
  step/1 -> S-Function Builder/4
  data/1 -> S-Function Builder/5
  data_length/1 -> S-Function Builder/6
  frameId_length/1 -> S-Function Builder/7

== system W01_Base_Map_cs/BMW_X5_SUV_1/ROS Send Camera 2/Image Publisher1 ==
  height : Inport
  width : Inport  Port=2
  encoding_length : Inport  Port=3
  step : Inport  Port=4
  data : Inport  Port=5
  data_length : Inport  Port=6
  frameId_length : Inport  Port=7
  S-Function Builder : S-Function  InitFcn=try, set_param(gcb,'FunctionName','Image_publisher'), end  FunctionName=Image_publisher  Parameters=int8(topic),int8(message_type),int8(frame_id),port,timeout  SFunctionModules=Image_publisher_wrapper rosbridge_functions  SFunctionDeploymentMode=off  EnableBusSupport=off  mask(S-Function Builder){}
      mask help: Simulink:masks:SFunctionBuilder_MD
      mask init: same as W01_Base_Map_cs/pose_otheCar/PoseArray Publisher/S-Function Builder
      settings: CopyFcn=set_param(gcbh,'LinkStatus','none')  PreSaveFcn=try, set_param(gcb,'FunctionName','Image_publisher'), end  OpenFcn=sfunctionwizard(gcbh)
      mask Display: plot(val(:,1),val(:,2)),disp(sys), port_label('input',1,'height'), port_label('input',2,'width'), port_label('input',3,'encoding_length'), port_label('input',4,'step'), port_label('input',5,'data'), port_label('input',6,'data_length'), port_label('input',7,'frameId_length')
  wires:
  height/1 -> S-Function Builder/1
  width/1 -> S-Function Builder/2
  encoding_length/1 -> S-Function Builder/3
  step/1 -> S-Function Builder/4
  data/1 -> S-Function Builder/5
  data_length/1 -> S-Function Builder/6
  frameId_length/1 -> S-Function Builder/7

== system W01_Base_Map_cs/BMW_X5_SUV_1/ROS Send Camera TL/Image Publisher1 ==
  height : Inport
  width : Inport  Port=2
  encoding_length : Inport  Port=3
  step : Inport  Port=4
  data : Inport  Port=5
  data_length : Inport  Port=6
  frameId_length : Inport  Port=7
  S-Function Builder : S-Function  InitFcn=try, set_param(gcb,'FunctionName','Image_publisher'), end  FunctionName=Image_publisher  Parameters=int8(topic),int8(message_type),int8(frame_id),port,timeout  SFunctionModules=Image_publisher_wrapper rosbridge_functions  SFunctionDeploymentMode=off  EnableBusSupport=off  mask(S-Function Builder){}
      mask help: Simulink:masks:SFunctionBuilder_MD
      mask init: same as W01_Base_Map_cs/pose_otheCar/PoseArray Publisher/S-Function Builder
      settings: CopyFcn=set_param(gcbh,'LinkStatus','none')  PreSaveFcn=try, set_param(gcb,'FunctionName','Image_publisher'), end  OpenFcn=sfunctionwizard(gcbh)
      mask Display: plot(val(:,1),val(:,2)),disp(sys), port_label('input',1,'height'), port_label('input',2,'width'), port_label('input',3,'encoding_length'), port_label('input',4,'step'), port_label('input',5,'data'), port_label('input',6,'data_length'), port_label('input',7,'frameId_length')
  wires:
  height/1 -> S-Function Builder/1
  width/1 -> S-Function Builder/2
  encoding_length/1 -> S-Function Builder/3
  step/1 -> S-Function Builder/4
  data/1 -> S-Function Builder/5
  data_length/1 -> S-Function Builder/6
  frameId_length/1 -> S-Function Builder/7

== system W01_Base_Map_cs/BMW_X5_SUV_1/ROS Send Clock/Clock Publisher ==
  secs : Inport
  nsecs : Inport  Port=2
  S-Function Builder : S-Function  InitFcn=try, set_param(gcb,'FunctionName','clock_publisher'), end  FunctionName=clock_publisher  Parameters=int8(topic),int8(message_type),port,timeout  SFunctionModules=clock_publisher_wrapper rosbridge_functions  SFunctionDeploymentMode=off  EnableBusSupport=off  mask(S-Function Builder){}
      mask help: Simulink:masks:SFunctionBuilder_MD
      mask init: same as W01_Base_Map_cs/pose_otheCar/PoseArray Publisher/S-Function Builder
      settings: CopyFcn=set_param(gcbh,'LinkStatus','none')  PreSaveFcn=try, set_param(gcb,'FunctionName','clock_publisher'), end  OpenFcn=sfunctionwizard(gcbh)
      mask Display: plot(val(:,1),val(:,2)),disp(sys), port_label('input',1,'secs'), port_label('input',2,'nsecs')
  wires:
  secs/1 -> S-Function Builder/1
  nsecs/1 -> S-Function Builder/2

== system W01_Base_Map_cs/BMW_X5_SUV_1/ROS Send GNSS/geometry_msgs//Pose ==
  positionX : Inport
  positionY : Inport  Port=2
  positionZ : Inport  Port=3
  orientationW : Inport  Port=4
  orientationX : Inport  Port=5
  orientationY : Inport  Port=6
  orientationZ : Inport  Port=7
  S-Function Builder1 : S-Function  InitFcn=try, set_param(gcb,'FunctionName','Pose_publisher'), end  FunctionName=Pose_publisher  Parameters=int8(topic),int8(message_type),port,timeout  SFunctionModules=Pose_publisher_wrapper rosbridge_functions  SFunctionDeploymentMode=off  EnableBusSupport=off  mask(S-Function Builder){}
      mask help: Simulink:masks:SFunctionBuilder_MD
      mask init: same as W01_Base_Map_cs/pose_otheCar/PoseArray Publisher/S-Function Builder
      settings: CopyFcn=set_param(gcbh,'LinkStatus','none')  PreSaveFcn=try, set_param(gcb,'FunctionName','Pose_publisher'), end  OpenFcn=sfunctionwizard(gcbh)
      mask Display: plot(val(:,1),val(:,2)),disp(sys), port_label('input',1,'positionX'), port_label('input',2,'positionY'), port_label('input',3,'positionZ'), port_label('input',4,'orientationW'), port_label('input',5,'orientationX'), port_label('input',6,'orientationY'), port_label('input',7,'orientationZ')
  wires:
  positionX/1 -> S-Function Builder1/1
  positionY/1 -> S-Function Builder1/2
  positionZ/1 -> S-Function Builder1/3
  orientationW/1 -> S-Function Builder1/4
  orientationX/1 -> S-Function Builder1/5
  orientationY/1 -> S-Function Builder1/6
  orientationZ/1 -> S-Function Builder1/7

== system W01_Base_Map_cs/BMW_X5_SUV_1/ROS Send Goal/geometry_msgs//PoseStamped ==
  seq : Inport
  frameId_length : Inport  Port=2
  Position.x : Inport  Port=3
  Position.y : Inport  Port=4
  Position.z : Inport  Port=5
  Orientation.w : Inport  Port=6
  Orientation.x : Inport  Port=7
  Orientation.y : Inport  Port=8
  Orientation.z : Inport  Port=9
  S-Function Builder1 : S-Function  InitFcn=try, set_param(gcb,'FunctionName','PoseStamped_publisher'), end  FunctionName=PoseStamped_publisher  Parameters=int8(topic),int8(message_type),port,timeout,uint8(1)  SFunctionModules=PoseStamped_publisher_wrapper rosbridge_functions  SFunctionDeploymentMode=off  EnableBusSupport=off  mask(S-Function Builder){}
      mask help: Simulink:masks:SFunctionBuilder_MD
      mask init: same as W01_Base_Map_cs/pose_otheCar/PoseArray Publisher/S-Function Builder
      settings: CopyFcn=set_param(gcbh,'LinkStatus','none')  PreSaveFcn=try, set_param(gcb,'FunctionName','PoseStamped_publisher'), end  OpenFcn=sfunctionwizard(gcbh)
      mask Display: plot(val(:,1),val(:,2)),disp(sys), port_label('input',1,'seq'), port_label('input',2,'frameId_length'), port_label('input',3,'positionX'), port_label('input',4,'positionY'), port_label('input',5,'positionZ'), port_label('input',6,'orientationW'), port_label('input',7,'orientationX'), port_label('input',8,'orientationY'), port_label('input',9,'orientationZ')
  wires:
  Position.x/1 -> S-Function Builder1/3
  Position.y/1 -> S-Function Builder1/4
  Position.z/1 -> S-Function Builder1/5
  Orientation.w/1 -> S-Function Builder1/6
  Orientation.x/1 -> S-Function Builder1/7
  Orientation.y/1 -> S-Function Builder1/8
  Orientation.z/1 -> S-Function Builder1/9
  seq/1 -> S-Function Builder1/1
  frameId_length/1 -> S-Function Builder1/2

== system W01_Base_Map_cs/BMW_X5_SUV_1/ROS Send IMU/sensor_msgs//Imu ==
  orientW : Inport
  orientX : Inport  Port=2
  orientY : Inport  Port=3
  orientZ : Inport  Port=4
  angularZ : Inport  Port=5
  linearAccX : Inport  Port=6
  linearAccZ : Inport  Port=7
  seq : Inport  Port=8
  frameId_length : Inport  Port=9
  S-Function Builder : S-Function  InitFcn=try, set_param(gcb,'FunctionName','Imu_publisher'), end  FunctionName=Imu_publisher  Parameters=int8(topic),int8(message_type),port,timeout  SFunctionModules=Imu_publisher_wrapper rosbridge_functions  SFunctionDeploymentMode=off  EnableBusSupport=off  mask(S-Function Builder){}
      mask help: Simulink:masks:SFunctionBuilder_MD
      mask init: same as W01_Base_Map_cs/pose_otheCar/PoseArray Publisher/S-Function Builder
      settings: CopyFcn=set_param(gcbh,'LinkStatus','none')  PreSaveFcn=try, set_param(gcb,'FunctionName','Imu_publisher'), end  OpenFcn=sfunctionwizard(gcbh)
      mask Display: plot(val(:,1),val(:,2)),disp(sys), port_label('input',1,'orientW'), port_label('input',2,'orientX'), port_label('input',3,'orientY'), port_label('input',4,'orientZ'), port_label('input',5,'angularZ'), port_label('input',6,'linearAccX'), port_label('input',7,'linearAccZ'), port_label('input',8,'seq'), port_label('input',9,'frameId_length')
  wires:
  orientW/1 -> S-Function Builder/1
  linearAccZ/1 -> S-Function Builder/7
  seq/1 -> S-Function Builder/8
  orientX/1 -> S-Function Builder/2
  orientY/1 -> S-Function Builder/3
  linearAccX/1 -> S-Function Builder/6
  frameId_length/1 -> S-Function Builder/9
  orientZ/1 -> S-Function Builder/4
  angularZ/1 -> S-Function Builder/5

== system W01_Base_Map_cs/BMW_X5_SUV_1/ROS Send Lidar/Float32MultiArray Publisher ==
  data : Inport
  size : Inport  Port=2
  S-Function Builder : S-Function  InitFcn=try, set_param(gcb,'FunctionName','Float32MultiArray_publisher'), end  FunctionName=Float32MultiArray_publisher  Parameters=int8(topic),int8(message_type),port,timeout  SFunctionModules=Float32MultiArray_publisher_wrapper rosbridge_functions  SFunctionDeploymentMode=off  EnableBusSupport=off  mask(S-Function Builder){}
      mask help: Simulink:masks:SFunctionBuilder_MD
      mask init: same as W01_Base_Map_cs/pose_otheCar/PoseArray Publisher/S-Function Builder
      settings: CopyFcn=set_param(gcbh,'LinkStatus','none')  PreSaveFcn=try, set_param(gcb,'FunctionName','Float32MultiArray_publisher'), end  OpenFcn=sfunctionwizard(gcbh)
      mask Display: plot(val(:,1),val(:,2)),disp(sys), port_label('input',1,'data'), port_label('input',2,'size')
  wires:
  data/1 -> S-Function Builder/1
  size/1 -> S-Function Builder/2

== system W01_Base_Map_cs/BMW_X5_SUV_1/ROS Send Odometry/nav_msgs//Odometry ==
  seq : Inport
  frameId_length : Inport  Port=2
  Pose : Inport  Port=3
  Velocity : Inport  Port=4
  linearY : Inport  Port=5
  linearZ : Inport  Port=6
  angularX : Inport  Port=7
  angularY : Inport  Port=8
  Yaw rate : Inport  Port=9
  Demux : Demux  Outputs=7
  S-Function Builder1 : S-Function  InitFcn=try, set_param(gcb,'FunctionName','Odometry_publisher'), end  FunctionName=Odometry_publisher  Parameters=int8(topic),int8(message_type),port,timeout  SFunctionModules=Odometry_publisher_wrapper rosbridge_functions  SFunctionDeploymentMode=off  EnableBusSupport=off  mask(S-Function Builder){}
      mask help: Simulink:masks:SFunctionBuilder_MD
      mask init: same as W01_Base_Map_cs/pose_otheCar/PoseArray Publisher/S-Function Builder
      settings: CopyFcn=set_param(gcbh,'LinkStatus','none')  PreSaveFcn=try, set_param(gcb,'FunctionName','Odometry_publisher'), end  OpenFcn=sfunctionwizard(gcbh)
      mask Display: plot(val(:,1),val(:,2)),disp(sys), port_label('input',1,'seq'), port_label('input',2,'frameId_length'), port_label('input',3,'childFrameId_length'), port_label('input',4,'positionX'), port_label('input',5,'positionY'), port_label('input',6,'positionZ'), port_label('input',7,'orientW'), port_label('input',8,'orientX'), port_label('input',9,'orientY'), port_label('input',10,'orientZ'), port_label('input',11,'linearX'), port_label('input',12,'linearY'), port_label('input',13,'linearZ'), port_label('input',14,'angularX'), port_label('input',15,'angularY'), port_label('input',16,'angularZ')
  wires:
  Demux/5 -> S-Function Builder1/8
  Pose/1 -> Demux/1
  Demux/4 -> S-Function Builder1/7
  Demux/7 -> S-Function Builder1/10
  Demux/1 -> S-Function Builder1/4
  Demux/2 -> S-Function Builder1/5
  Demux/3 -> S-Function Builder1/6
  Demux/6 -> S-Function Builder1/9
  Velocity/1 -> S-Function Builder1/11
  Yaw rate/1 -> S-Function Builder1/16
  seq/1 -> S-Function Builder1/1
  frameId_length/1 -> S-Function Builder1/3, S-Function Builder1/2
  linearY/1 -> S-Function Builder1/12
  linearZ/1 -> S-Function Builder1/13
  angularX/1 -> S-Function Builder1/14
  angularY/1 -> S-Function Builder1/15
